simulink model "bench_string_heat"  (R2024b)
settings: Solver=daessc  StartTime=0.0  StopTime=300  MaxStep=1  RelTol=1e-3
values from neighbouring files (symbols this model uses):
  PN = evalin('base','PN')    [run_bench_string_heat.m]
undefined symbols (not defined in the file or in its folder): T_bench
libraries: fl_lib x2, nesl_utility x2, loco_native_lib x1
settings Model: Creator=BillBeverley  LastModifiedBy=BillBeverley

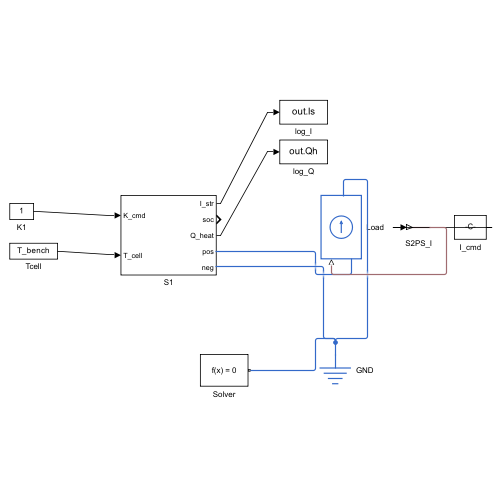
[thumbnail: Simulink's stored preview of the top-level diagram]
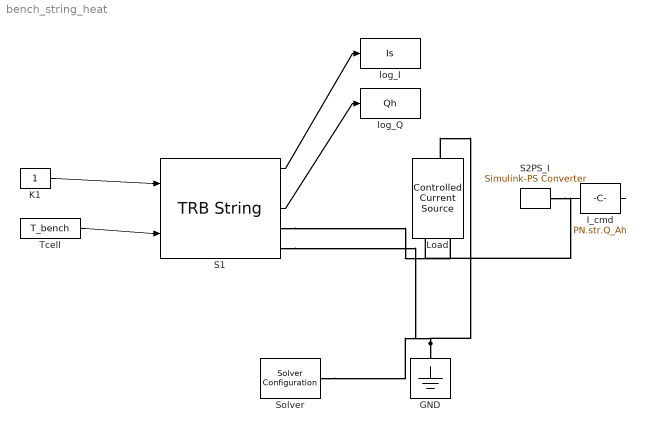
== system bench_string_heat ==
  GND : fl_lib/Electrical/Electrical Elements/Electrical Reference
  I_cmd : Constant  Value=PN.str.Q_Ah
  K1 : Constant
  Load : fl_lib/Electrical/Electrical Sources/Controlled Current Source
  S1 : loco_native_lib/TRB String  SystemSampleTime=-1  VariantActivationTime=update diagram  AllowFlexibleInterface=on  Latency=0  AutoFrameSizeCalculation=off
  S2PS_I : nesl_utility/Simulink-PS Converter  PhysicalDomain=network_engine_domain  SubClassName=ps_input  LeftPortType=input  RightPortType=output  PseudoPeriodic=off  Frequencies=[]  NoiseDistribution=none  NoiseParameters=[]  Unit=A  AffineConversion=off  FilteringAndDerivatives=provide  SimscapeFilterOrder=1  InputFilterTimeConstant=0.001  UdotUserProvided=0
  Solver : nesl_utility/Solver Configuration  PhysicalDomain=network_engine_domain  SubClassName=solver  LeftPortType=input  RightPortType=generic  Tones=[]  Harmonics=[]  SimulateNoise=off  Profile=off  UseLocalSampling=off  EnableSwitchedLinearOptims=on  FrequencyDomain=off  UseCCode=off  RelTol=0.001  AbsTol=0.001  MinStep=1e-09  ToWorkspace=off  RevertToSquareIcSolve=off  NumHomotopyIterations=100  PhasorMode=off  PhasorModeNumHarmonics=1  ConsistencySolver=NEWTON_XTOL_AFTER_FTOL  IndexReductionMethod=DerivativeReplacement  DoDC=off  ResidualTolerance=1e-09  ConsistencyTolSource=GLOBAL  ConsistencyAbsTol=0.001  ConsistencyRelTol=0.001  ConsistencyTolFactor=0.001  UseLocalSolver=off  LocalSolverChoice=NE_BACKWARD_EULER_ADVANCER  ResolveIndetEquations=on  FunctionEvalNumThread=1  LocalSolverSampleTime=0.001  DoFixedCost=off  MaxNonlinIter=3  MaxModeIter=2  ComputeImpulses=off  ImpulseIterations=2  LinearAlgebra=auto  LinearAlgebraNumThread=0  EquationFormulation=NE_TIME_EF  DelaysMemoryBudget=1024  AutomaticFiltering=on  FilteringTimeConstant=0.001  PartitionStorageMethod=AS_NEEDED  PartitionMemoryBudget=1024  PartitionMethod=ROBUST  MultibodyUseLocalSolver=off  MultibodyLocalSolverChoice=ODE1  MultibodyLocalSolverSampleTime=0.001
  Tcell : Constant  Value=T_bench
  log_I : ToWorkspace  VariableName=Is  SaveFormat=Timeseries  SampleTime=-1
  log_Q : ToWorkspace  VariableName=Qh  SaveFormat=Timeseries  SampleTime=-1
  wires:
  K1/1 -> S1/1
  Tcell/1 -> S1/2
  S1/3 -> log_Q/1
  S1/1 -> log_I/1
  I_cmd/1 -> S2PS_I/1
  connections:
  S1/RConn1 -- Load/RConn2
  Load/LConn1 -- S1/RConn2 -- GND/LConn1 -- Solver/RConn1
  S2PS_I/RConn1 -- Load/RConn1
